simulink model "AR_Drone_Mission_Height"  (R2014a)
settings: configuration reference "AR_Drone_ConfigSet_NOEXT" (kept outside this file)
settings Model: SimulationMode=external  ExtModeTrigDuration=48000  Creator=nraman  LastModifiedBy=Raphaël

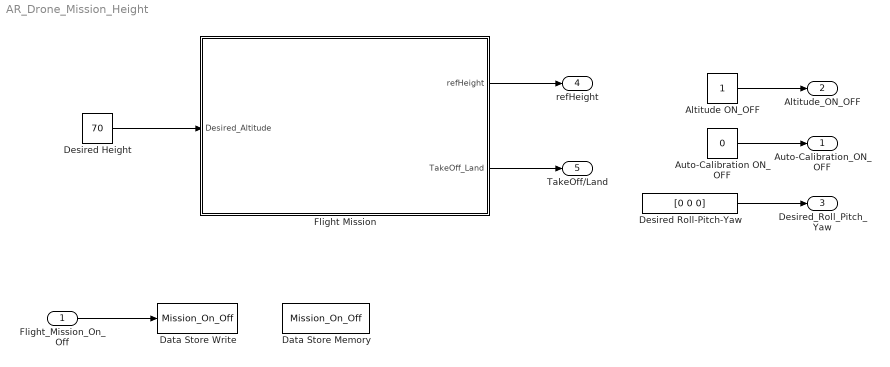
== system AR_Drone_Mission_Height ==
  Flight_Mission_On_Off : Inport
  Altitude ON_OFF : Constant
  Auto-Calibration ON_OFF : Constant  Value=0
  Data Store Memory : DataStoreMemory  DataStoreName=Mission_On_Off  ReadBeforeWriteMsg=warning  WriteAfterWriteMsg=warning  WriteAfterReadMsg=warning  OutDataTypeStr=boolean
  Data Store Write : DataStoreWrite  DataStoreName=Mission_On_Off
  Desired Height : Constant  Value=70
  Desired Roll-Pitch-Yaw : Constant  Value=[0 0 0]
  Flight Mission : Stateflow chart  TreatAsAtomicUnit=on
  Auto-Calibration_ON_OFF : Outport  PortDimensions=1
  Altitude_ON_OFF : Outport  Port=2  PortDimensions=1
  Desired_Roll_Pitch_Yaw : Outport  Port=3  PortDimensions=3
  refHeight : Outport  Port=4  PortDimensions=1
  TakeOff/Land : Outport  Port=5  PortDimensions=1
  wires:
  Flight_Mission_On_Off/1 -> Data Store Write/1
  Flight Mission/1(refHeight) -> refHeight/1
  Desired Height/1 -> Flight Mission/1(Desired_Altitude)
  Desired Roll-Pitch-Yaw/1 -> Desired_Roll_Pitch_Yaw/1
  Altitude ON_OFF/1 -> Altitude_ON_OFF/1
  Auto-Calibration ON_OFF/1 -> Auto-Calibration_ON_OFF/1
  Flight Mission/2(TakeOff_Land) -> TakeOff/Land/1

== stateflow chart AR_Drone_Mission_Height/Flight Mission ==
  state Algorithm_Choice [parallel]
    settings: executionOrder=1
    state Do_Nothing
      entry:
      refHeight = 0;
      TakeOff_Land = 0;
    state Flight_Mission
      entry : TakeOff_Land = 0 ;
      note: Description:
          | -Upon entry, this block will set the motor to ARMED (enable controller integrator and motor safetey unclamped)
          | -This block will command the AR Drone to fly up to a certain height using the variable refHeight
          | -The output of refHeight should be a function of desired Altitude. The most primitive assignment is to make refHeight = DesiredAltitude, this is comparable to giving the drone a step response. Alternate methods could be giving it a smooth trajectory to follow from the ground to that particular height
          |
          | -Below is an example of what it might look like
      state Altitude_Climb
        entry,during: refHeight = Desired_Altitude;
      state Land
        entry: TakeOff_Land = -1;
      (default) -> Altitude_Climb
      Altitude_Climb -> Land : after(2,sec)
    (default) -> Algorithm_Choice.Do_Nothing
    Algorithm_Choice.Do_Nothing -> Flight_Mission : [Mission_On_Off == true]
    Flight_Mission -> Algorithm_Choice.Do_Nothing : [Mission_On_Off == false]
  state Launch_Mission [parallel]
    settings: executionOrder=2
    state Do_Nothing
      entry: TakeOff_Land = 0;
    state Take_Off
      entry: TakeOff_Land = 1;
    (default) -> Launch_Mission.Do_Nothing
    Launch_Mission.Do_Nothing -> Take_Off : after(5,sec)
  data: Desired_Altitude input; refHeight output; Mission_On_Off data_store_memory; TakeOff_Land output
  data refHeight settings: description=Desired height at which the drone needs to hover.
